simulink model "Vehicle3DOFModel"  (R2018a)
settings: Solver=VariableStepAuto  StartTime=0.0  StopTime=10.0  RelTol=1e-3
undefined symbols (not defined in the file): Cf, Cr, Iz, lf, lr, m, tau, v0_ego
settings Model: Creator=CHIZOM WORNU  LastModifiedBy=CHIZOM WORNU

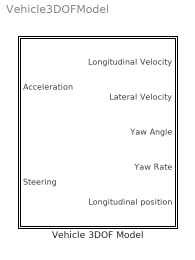
== system Vehicle3DOFModel ==
  "  Vehicle 3DOF Model " : Subsystem

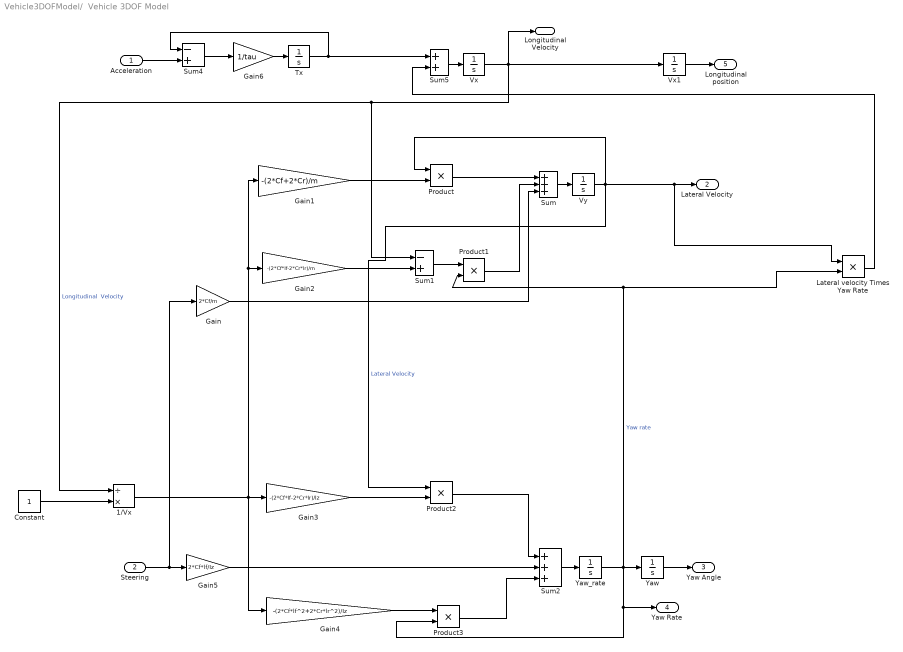
== system Vehicle3DOFModel/  Vehicle 3DOF Model  ==
  Acceleration : Inport
  Steering : Inport  Port=2
  1/Vx : Product  Inputs=/*
  Constant : Constant
  Gain : Gain  Gain=2*Cf/m
  Gain1 : Gain  Gain=-(2*Cf+2*Cr)/m
  Gain2 : Gain  Gain=-(2*Cf*lf-2*Cr*lr)/m
  Gain3 : Gain  Gain=-(2*Cf*lf-2*Cr*lr)/Iz
  Gain4 : Gain  Gain=-(2*Cf*lf^2+2*Cr*lr^2)/Iz
  Gain5 : Gain  Gain=2*Cf*lf/Iz
  Gain6 : Gain  Gain=1/tau
  Lateral velocity Times Yaw Rate : Product
  Product{,1..3} (4 alike) : Product
  Sum : Sum  Inputs=+++
  Sum1 : Sum  Inputs=-+
  Sum2 : Sum  Inputs=+++
  Sum4 : Sum  Inputs=-+
  Sum5 : Sum
  Tx : Integrator
  Vx : Integrator  InitialCondition=v0_ego
  Vx1 : Integrator  InitialCondition=v0_ego
  Vy : Integrator
  Yaw : Integrator
  "Yaw_rate " : Integrator
  Longitudinal Velocity : Outport
  Lateral Velocity : Outport  Port=2
  Yaw Angle : Outport  Port=3
  Yaw Rate : Outport  Port=4
  Longitudinal position : Outport  Port=5
  wires:
  Vx/1 -> Sum1/1, 1/Vx/1, Vx1/1, Longitudinal Velocity/1  "Longitudinal  Velocity"
  Vy/1 -> Product2/1, Product/1, Lateral velocity Times Yaw Rate/1, Lateral Velocity/1  "Lateral Velocity"
  Yaw/1 -> Yaw Angle/1
  "Yaw_rate "/1 -> Yaw/1, Yaw Rate/1, Product3/2, Lateral velocity Times Yaw Rate/2, Product1/2  "Yaw rate"
  Vx1/1 -> Longitudinal position/1
  Product1/1 -> Sum/2
  Sum/1 -> Vy/1
  Product/1 -> Sum/1
  Gain1/1 -> Product/2
  Steering/1 -> Gain/1, Gain5/1
  Gain/1 -> Sum/3
  Sum1/1 -> Product1/1
  Lateral velocity Times Yaw Rate/1 -> Sum5/2
  Gain5/1 -> Sum2/2
  Product3/1 -> Sum2/3
  Tx/1 -> Sum5/1, Sum4/1
  Acceleration/1 -> Sum4/2
  Sum4/1 -> Gain6/1
  Product2/1 -> Sum2/1
  1/Vx/1 -> Gain4/1, Gain3/1, Gain1/1, Gain2/1
  Gain3/1 -> Product2/2
  Constant/1 -> 1/Vx/2
  Gain4/1 -> Product3/1
  Gain2/1 -> Sum1/2
  Sum5/1 -> Vx/1
  Sum2/1 -> "Yaw_rate "/1
  Gain6/1 -> Tx/1
